simulink model "test_polbereichsvorgabe"  (R2016b)
settings: Solver=FixedStepAuto  StartTime=0.0  StopTime=20.0  FixedStep=1e-3  RelTol=1e-3
values from neighbouring files (symbols this model uses):
  A_D = -x(8)    [calc_regler_polbereichsvorgabe.m]
  B_D = [-x(5), -x(6), -x(7)]    [calc_regler_polbereichsvorgabe.m]
  C_D = x(4)    [calc_regler_polbereichsvorgabe.m]
  D_D = [x(1), x(2), x(3)]    [calc_regler_polbereichsvorgabe.m]
undefined symbols (not defined in the file or in its folder): system
settings Model: Creator=nicol  LastModifiedBy=nicol

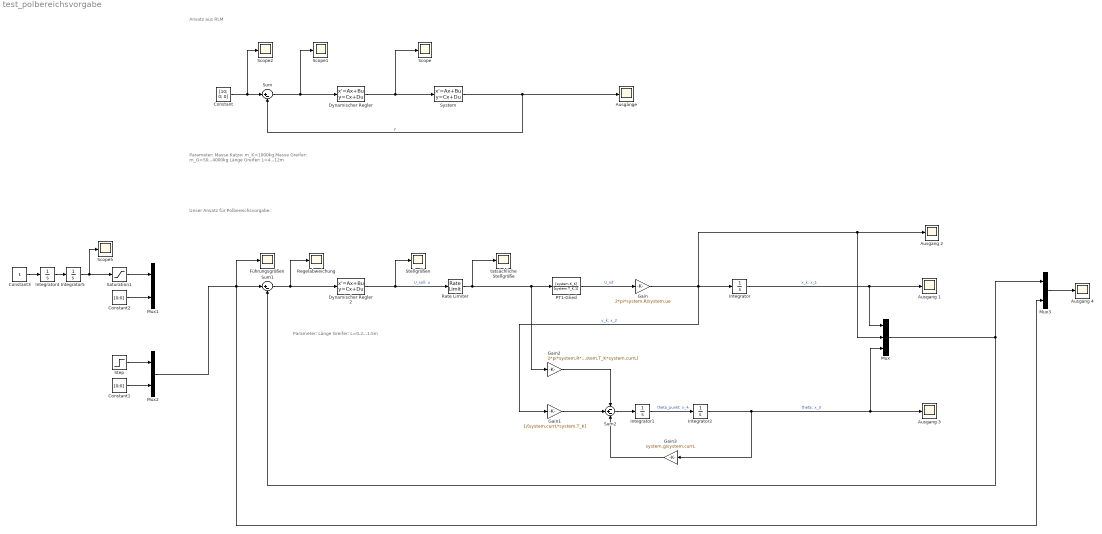
== system test_polbereichsvorgabe ==
  note: Ansatz aus RLM
  note: Parameter:
      | Masse Katze: m_K=1000kg
      | Masse Greifer: m_G=50...4000kg
      | Länge Greifer: L=4...12m
  note: Unser Ansatz für Polbereichsvorgabe:
  note: Parameter:
      | Länge Greifer: L=0.2...1.5m
  Ausgang {1..4} (4 alike) : Scope
  Ausgänge : Scope
  Constant : Constant  Value=[10; 0; 0]  VectorParams1D=off
  Constant1 : Constant  Value=[0;0]  VectorParams1D=off
  Constant2 : Constant  Value=[0;0]  VectorParams1D=off
  Constant3 : Constant
  Dynamischer Regler : StateSpace  A=-0.6  B=[7.2 25.4 -306.2]  C=1000.7  D=[144.7 10294.8 -10032.5]  X0=0
  Dynamischer Regler 2 : StateSpace  A=A_D  B=-B_D  C=-C_D  D=D_D  X0=0
  Führungsgrößen : Scope
  Gain : Gain  Gain=2*pi*system.R/system.ue
  Gain1 : Gain  Gain=1/(system.currL*system.T_K)
  Gain2 : Gain  Gain=2*pi*system.R*system.K_K/(system.ue*system.T_K*system.currL)
  Gain3 : Gain  Gain=system.g/system.currL
  Integrator{,1..2,4..5} (5 alike) : Integrator
  Mux : Mux  Inputs=3
  Mux1 : Mux  Inputs=2
  Mux2 : Mux  Inputs=2
  Mux3 : Mux  Inputs=2
  PT1-Glied : TransferFcn  Numerator=[system.K_K]  Denominator=[system.T_K,1]
  Rate Limiter : RateLimiter  RisingSlewLimit=4.32  FallingSlewLimit=-4.32  SampleTimeMode=inherited
  Regelabweichung : Scope
  Saturation1 : Saturate  UpperLimit=2  LowerLimit=-2
  Scope{,1..2,5} (4 alike) : Scope
  Stellgrößen : Scope
  Step : Step  After=2  SampleTime=0
  Sum : Sum  Inputs=|+-
  Sum1 : Sum  Inputs=|+-
  Sum2 : Sum  Inputs=-+-
  System : StateSpace  A=[0 1 0 0; 0 0 39.24 0; 0 0 0 1; 0 0 -4.0875 0]  B=[0; 0.001; 0; -0.000083333]  C=[1 0 0 0; 0 1 0 0; 0 0 1 0]  D=[0; 0; 0]  X0=0
  tatsächliche Stellgröße : Scope
  wires:
  System/1 -> Sum/2, Ausgänge/1  "y"
  Constant/1 -> Scope2/1, Sum/1
  Dynamischer Regler/1 -> Scope/1, System/1
  Sum/1 -> Scope1/1, Dynamischer Regler/1
  Sum1/1 -> Dynamischer Regler 2/1, Regelabweichung/1
  PT1-Glied/1 -> Gain/1  "U_ist"
  Gain/1 -> Mux/2, Ausgang 2/1, Integrator/1, Gain1/1  "v_k; x_2"
  Integrator/1 -> Mux/1, Ausgang 1/1  "x_k; x_1"
  Gain2/1 -> Sum2/1
  Sum2/1 -> Integrator1/1
  Integrator1/1 -> Integrator2/1  "theta_punkt; x_4"
  Integrator2/1 -> Gain3/1, Mux/3, Ausgang 3/1  "theta; x_3"
  Gain3/1 -> Sum2/3
  Gain1/1 -> Sum2/2
  Dynamischer Regler 2/1 -> Rate Limiter/1, Stellgrößen/1  "U_soll; u"
  Mux/1 -> Mux3/1, Sum1/2
  Integrator4/1 -> Integrator5/1
  Integrator5/1 -> Saturation1/1, Scope5/1
  Constant3/1 -> Integrator4/1
  Saturation1/1 -> Mux1/1
  Constant2/1 -> Mux1/2
  Mux2/1 -> Mux3/2, Führungsgrößen/1, Sum1/1
  Constant1/1 -> Mux2/2
  Step/1 -> Mux2/1
  Rate Limiter/1 -> PT1-Glied/1, Gain2/1, tatsächliche Stellgröße/1
  Mux3/1 -> Ausgang 4/1
